simulink model "full_simulation_split_hil_new_connection"  (Simulink 7.9)
settings: Solver=ode1  StartTime=0  StopTime=10  FixedStep=Ts  RelTol=1e-8
values from neighbouring files (symbols this model uses):
  A_fx = 2e-2 * 0.4    (= 0.008)    [QR_DI_Init.m]    (also in quadro_cascade_disturbance_wo_wind.m)
  A_fy = A_fx    (= 0.008)    [QR_DI_Init.m]    (also in quadro_cascade_disturbance_wo_wind.m)
  A_fz = 2 * A_fx    (= 0.016)    [QR_DI_Init.m]    (also in quadro_cascade_disturbance_wo_wind.m)
  Bias_Phi = -0.0088    [QR_DI_Init.m]    (also in Reference_Calibration.m = mean(Phi))
  Bias_Theta = 0.022    [QR_DI_Init.m]    (also in Reference_Calibration.m = mean(Theta))
  command_on = 1    [QR_DI_Init.m]    (also in quadro_cascade_disturbance_wo_wind.m)
  cw_x = 1.05    [QR_DI_Init.m]    (also in quadro_cascade_disturbance_wo_wind.m)
  cw_y = cw_x    (= 1.05)    [QR_DI_Init.m]    (also in quadro_cascade_disturbance_wo_wind.m)
  cw_z = 1.05    [QR_DI_Init.m]    (also in quadro_cascade_disturbance_wo_wind.m)
  deltaTm = 0.2    [QR_DI_Init.m]    (also in quadro_cascade_disturbance_wo_wind.m)
  den_psi_ref = poly( ones(1,2) * -1 * T_psi_ref)    [QR_DI_Init.m]    (also in quadro_cascade_disturbance_wo_wind.m)
  den_x_ref = poly( ones(1,4) * -1 * T_x_ref)    [QR_DI_Init.m]    (also in quadro_cascade_disturbance_wo_wind.m)
  den_y_ref = poly( ones(1,4) * -1 * T_y_ref)    [QR_DI_Init.m]    (also in quadro_cascade_disturbance_wo_wind.m)
  den_z_ref = poly( ones(1,4) * -1 * T_z_ref)    [QR_DI_Init.m]    (also in quadro_cascade_disturbance_wo_wind.m)
  drot = 0.0117    [QR_DI_Init.m]    (also in quadro_cascade_disturbance_wo_wind.m = 0.2)
  dtran = 0.01    [QR_DI_Init.m]    (also in quadro_cascade_disturbance_wo_wind.m = 0.003)
  Fz_gain = 1 + 0.05*rand(1)    [QR_DI_Init.m]    (also in quadro_cascade_disturbance_wo_wind.m)
  Fz_lo = - 1.2 * m * g    (= -3.5316)    [QR_DI_Init.m]    (also in quadro_cascade_disturbance_wo_wind.m = -4.1202)
  Fz_up = 0    [QR_DI_Init.m]    (also in quadro_cascade_disturbance_wo_wind.m)
  g = 9.81    [QR_DI_Init.m]    (also in quadro_cascade_disturbance_wo_wind.m)
  Iq = [I_xx 0 0 ; 0 I_yy 0 ; 0 0 I_zz ]    [QR_DI_Init.m]    (also in quadro_cascade_disturbance_wo_wind.m = [0.0605 0 0; 0 0.0605 0; 0 0 0.018])
  K_err = old(:,2:end)    [QR_DI_Init.m]    (also in quadro_cascade_disturbance_wo_wind.m)
  K_Mot_Force = 0.3512    [QR_DI_Init.m]    (also in quadro_cascade_disturbance_wo_wind.m)
  K_Mot_Torque = 0.013    [QR_DI_Init.m]    (also in quadro_cascade_disturbance_wo_wind.m = 0.0013)
  l = 0.25    [QR_DI_Init.m]    (also in quadro_cascade_disturbance_wo_wind.m = 0.2775)
  m = 0.30    (= 0.3)    [QR_DI_Init.m]    (also in quadro_cascade_disturbance_wo_wind.m)
  m_real = m * ( 1 + 0.05*rand(1))    [QR_DI_Init.m]    (also in quadro_cascade_disturbance_wo_wind.m)
  Mm = 0.0    (= 0)    [QR_DI_Init.m]    (also in quadro_cascade_disturbance_wo_wind.m = 0.5)
  Mx_lo = - Mx_up    (= -0.2)    [QR_DI_Init.m]    (also in quadro_cascade_disturbance_wo_wind.m)
  Mx_up = 0.20    (= 0.2)    [QR_DI_Init.m]    (also in quadro_cascade_disturbance_wo_wind.m)
  My_lo = - My_up    (= -0.2)    [QR_DI_Init.m]    (also in quadro_cascade_disturbance_wo_wind.m)
  My_up = 0.20    (= 0.2)    [QR_DI_Init.m]    (also in quadro_cascade_disturbance_wo_wind.m)
  Mz_lo = - Mz_up    (= -0.02)    [QR_DI_Init.m]    (also in quadro_cascade_disturbance_wo_wind.m = -0.002)
  Mz_up = 0.02    [QR_DI_Init.m]    (also in quadro_cascade_disturbance_wo_wind.m = 0.002)
  phase_wind_z = 0    [QR_DI_Init.m]    (also in quadro_cascade_disturbance_wo_wind.m)
  psi_p_lim = 10*pi/180    (= 0.174532925199)    [QR_DI_Init.m]    (also in quadro_cascade_disturbance_wo_wind.m = 5)
  PWM_MAX = 200    [QR_DI_Init.m]    (also in quadro_cascade_disturbance_wo_wind.m)
  rho_air = 1.2041    [QR_DI_Init.m]    (also in quadro_cascade_disturbance_wo_wind.m)
  sample_time_noise_psi = 0.1    [QR_DI_Init.m]
  sample_time_noise_x = 0.2    [QR_DI_Init.m]
  sample_time_noise_y = 0.2    [QR_DI_Init.m]
  sample_time_noise_z = 0.1    [QR_DI_Init.m]
  seed_psi = seedvector(7)    [QR_DI_Init.m]
  seed_x = seedvector(1)    [QR_DI_Init.m]    (also in quadro_cascade_disturbance_wo_wind.m)
  seed_xp = seedvector(4)    [QR_DI_Init.m]    (also in quadro_cascade_disturbance_wo_wind.m)
  seed_y = seedvector(2)    [QR_DI_Init.m]    (also in quadro_cascade_disturbance_wo_wind.m)
  seed_yp = seedvector(5)    [QR_DI_Init.m]    (also in quadro_cascade_disturbance_wo_wind.m)
  seed_z = seedvector(3)    [QR_DI_Init.m]    (also in quadro_cascade_disturbance_wo_wind.m)
  seed_zp = seedvector(6)    [QR_DI_Init.m]    (also in quadro_cascade_disturbance_wo_wind.m)
  std_dev_psi = 1 * pi/180 * Noise_on    (= 0)    [QR_DI_Init.m]
  std_dev_x = 1e-1 * Noise_on    (= 0)    [QR_DI_Init.m]
  std_dev_xp = 0.03 * Noise_on    (= 0)    [QR_DI_Init.m]
  std_dev_y = 1e-1 * Noise_on    (= 0)    [QR_DI_Init.m]
  std_dev_yp = 0.03 * Noise_on    (= 0)    [QR_DI_Init.m]
  std_dev_z = 0.03 * Noise_on    (= 0)    [QR_DI_Init.m]
  std_dev_zp = 0.03 * Noise_on    (= 0)    [QR_DI_Init.m]
  T_refalt = 0.01    [QR_DI_Init.m]    (also in quadro_cascade_disturbance_wo_wind.m)
  T_wind_z = 24    [QR_DI_Init.m]    (also in quadro_cascade_disturbance_wo_wind.m)
  Tm = 10    [QR_DI_Init.m]    (also in quadro_cascade_disturbance_wo_wind.m)
  Ts = 1e-2    (= 0.01)    [QR_DI_Init.m]    (also in quadro_cascade_disturbance_wo_wind.m)
  v_wind_max_z = 2    [QR_DI_Init.m]    (also in quadro_cascade_disturbance_wo_wind.m)
  wind_on = 0    [QR_DI_Init.m]    (also in quadro_cascade_disturbance_wo_wind.m)
  x_p_lim = 1.5    [QR_DI_Init.m]    (also in quadro_cascade_disturbance_wo_wind.m = 5)
  y_p_lim = 1.5    [QR_DI_Init.m]    (also in quadro_cascade_disturbance_wo_wind.m = 5)
  z_p_lim = 1    [QR_DI_Init.m]    (also in quadro_cascade_disturbance_wo_wind.m = 1.5)
undefined symbols (not defined in the file or in its folder): T_wind_fine, v_wind_x_fine, v_wind_y_fine
libraries: simulink x5, dspsigops x4, Ports x4, aerolibtransform2 x3, dspmtrx3 x1, aerolibutil x1
(part 2 of 6)

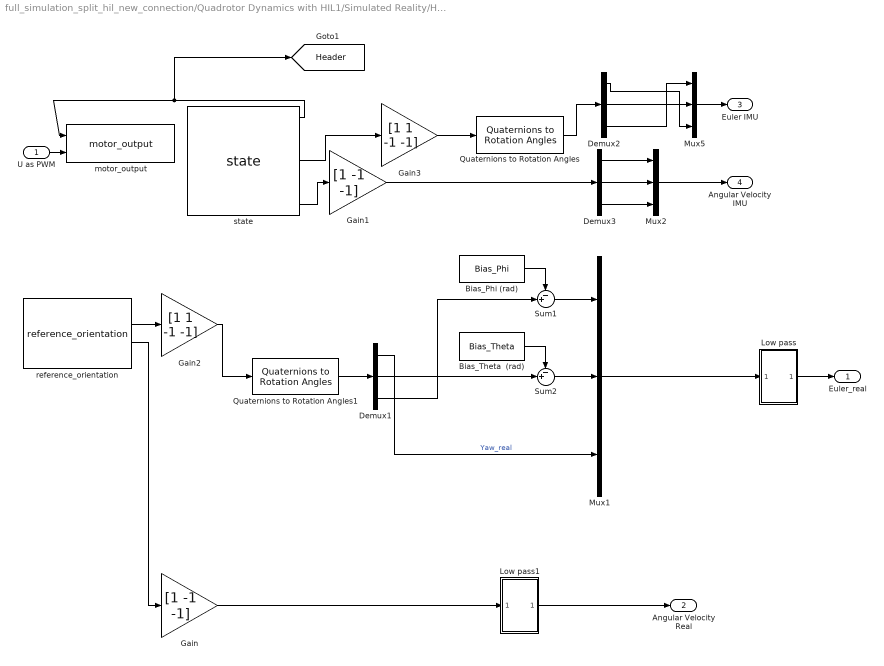
== system full_simulation_split_hil_new_connection/Quadrotor Dynamics with HIL1/Simulated Reality/HIL in the Loop for Rotation/Test Rig ==
  U as PWM : Inport
  Bias_Phi (rad) : Constant  Value=Bias_Phi
  Bias_Theta  (rad) : Constant  Value=Bias_Theta
  Demux1 : Demux  Outputs=3
  Demux2 : Demux  Outputs=3
  Demux3 : Demux  Outputs=3
  Gain : Gain  Gain=[1 -1 -1]
  Gain1 : Gain  Gain=[1 -1 -1]
  Gain2 : Gain  Gain=[1 1 -1 -1]
  Gain3 : Gain  Gain=[1 1 -1 -1]
  Low pass : Subsystem  mask{T_refalt=T_refalt}
  Low pass1 : Subsystem  mask{T_refalt=T_refalt}
  Mux1 : Mux  Inputs=3
  Mux2 : Mux  Inputs=3
  Mux5 : Mux  Inputs=3
  Quaternions to Rotation Angles : aerolibtransform2/Quaternions to Rotation Angles  rotationOrder=ZYX
  Quaternions to Rotation Angles1 : aerolibtransform2/Quaternions to Rotation Angles  rotationOrder=ZYX
  Sum1 : Sum  Inputs=-+|
  Sum2 : Sum  Inputs=-+|
  motor_output : Ports/motor_output
  reference_orientation : Ports/reference_orientation
  state : Ports/state
  "Euler_real " : Outport
  Angular Velocity Real : Outport  Port=2
  Euler IMU : Outport  Port=3
  Angular Velocity IMU : Outport  Port=4
  tag scope: Header=global
  wires:
  U as PWM/1 -> motor_output/2
  Mux5/1 -> Euler IMU/1
  Low pass/1(Out1) -> "Euler_real "/1
  state/1 -> motor_output/1, [Header]
  state/3 -> Gain3/1
  Quaternions to Rotation Angles/1 -> Demux2/1
  Demux2/2 -> Mux5/2
  Demux2/3 -> Mux5/1
  state/5 -> Gain1/1
  reference_orientation/2 -> Gain2/1
  reference_orientation/3 -> Gain/1
  Low pass1/1(Out1) -> Angular Velocity Real/1
  Gain2/1 -> Quaternions to Rotation Angles1/1
  Gain3/1 -> Quaternions to Rotation Angles/1
  Demux1/1 -> Mux1/3  "Yaw_real"
  Demux1/2 -> Sum2/2
  Quaternions to Rotation Angles1/1 -> Demux1/1
  Mux1/1 -> Low pass/1(In1)
  Gain/1 -> Low pass1/1(In1)
  Gain1/1 -> Demux3/1
  Demux3/1 -> Mux2/1
  Demux3/2 -> Mux2/2
  Mux2/1 -> Angular Velocity IMU/1
  Demux3/3 -> Mux2/3
  Demux2/1 -> Mux5/3
  Sum1/1 -> Mux1/1
  Sum2/1 -> Mux1/2
  Demux1/3 -> Sum1/2
  Bias_Phi (rad)/1 -> Sum1/1
  Bias_Theta  (rad)/1 -> Sum2/1

== system full_simulation_split_hil_new_connection/Quadrotor Dynamics with HIL1/Simulated Reality/Translation of the Quadrotor/transform to Inertial axes  ==
  x y z : Inport
  transform coefficients : Inport  Port=2
  Product : Product  Multiplication=Matrix(*)  SaturateOnIntegerOverflow=on  InputSameDT=on  OutDataTypeStr=Inherit: Same as first input
  Ve : Outport
  wires:
  x y z/1 -> Product/2
  transform coefficients/1 -> Product/1
  Product/1 -> Ve/1

== system full_simulation_split_hil_new_connection/Quadrotor Dynamics with HIL1/Simulated Reality/HIL in the Loop for Rotation/Test Rig/Low pass ==
  In1 : Inport
  Demux3 : Demux  Outputs=3
  Mux1 : Mux  Inputs=3
  Transfer Fcn1 : TransferFcn  Denominator=[T_refalt 1]
  Transfer Fcn2 : TransferFcn  Denominator=[T_refalt 1]
  Transfer Fcn3 : TransferFcn  Denominator=[T_refalt 1]
  Out1 : Outport
  wires:
  Demux3/1 -> Transfer Fcn1/1
  Transfer Fcn1/1 -> Mux1/1
  Demux3/2 -> Transfer Fcn2/1
  Transfer Fcn2/1 -> Mux1/2
  Demux3/3 -> Transfer Fcn3/1
  Transfer Fcn3/1 -> Mux1/3
  In1/1 -> Demux3/1
  Mux1/1 -> Out1/1

== system full_simulation_split_hil_new_connection/Quadrotor Dynamics with HIL1/Simulated Reality/HIL in the Loop for Rotation/Test Rig/Low pass1 ==
  In1 : Inport
  Demux3 : Demux  Outputs=3
  Mux1 : Mux  Inputs=3
  Transfer Fcn1 : TransferFcn  Denominator=[T_refalt 1]
  Transfer Fcn2 : TransferFcn  Denominator=[T_refalt 1]
  Transfer Fcn3 : TransferFcn  Denominator=[T_refalt 1]
  Out1 : Outport
  wires:
  Mux1/1 -> Out1/1
  In1/1 -> Demux3/1
  Transfer Fcn3/1 -> Mux1/3
  Demux3/3 -> Transfer Fcn3/1
  Transfer Fcn2/1 -> Mux1/2
  Demux3/2 -> Transfer Fcn2/1
  Transfer Fcn1/1 -> Mux1/1
  Demux3/1 -> Transfer Fcn1/1

== matlab function Dynamic Inversion of the Extended System/invAx SH/Embedded MATLAB Function ==
  data: xwhole_ext input double size=[14 1]; invAx output double size=[4 4]; m input double; I input double size=[3 3]; dtran input double; drot input double; Ax output double
function [invAx, Ax] = fcn(xwhole_ext, m, I, dtran, drot)
% This block supports the Embedded MATLAB subset.
% See the help menu for details. 
x = xwhole_ext(1);
y = xwhole_ext(2);
z = xwhole_ext(3);
dx = xwhole_ext(4);
dy = xwhole_ext(5);
dz = xwhole_ext(6);

phi = xwhole_ext(7);
theta = xwhole_ext(8);
psi = xwhole_ext(9);
p = xwhole_ext(10);
q = xwhole_ext(11);
r = xwhole_ext(12);

xi1 = xwhole_ext(13) +eps;
dxi1 = xwhole_ext(14) +eps;




% g = -9.81;  % not needed, S.H. 26.03.2013


Ixx = I(1,1);
Ixy = I(1,2);
Ixz = I(1,3);
Iyy = I(2,2);
Iyz = I(2,3);
Izz = I(3,3);

% invAx =[ ...
% (sin(phi)*sin(psi)*sin(theta)^2+cos(psi)*cos(phi)*sin(theta)+sin(psi)*cos(theta)^2*sin(phi))*m/(sin(psi)^2*sin(phi)^2*sin(theta)^2+sin(psi)^2*sin(phi)^2*cos(theta)^2+cos(psi)^2*cos(phi)^2*sin(theta)^2+cos(phi)^2*sin(psi)^2*sin(theta)^2+cos(psi)^2*sin(phi)^2*sin(theta)^2+cos(psi)^2*sin(phi)^2*cos(theta)^2+cos(theta)^2*cos(phi)^2*sin(psi)^2+cos(theta)^2*cos(phi)^2*cos(psi)^2),          -(-cos(phi)*sin(psi)*sin(theta)+cos(psi)*sin(phi)*sin(theta)^2+cos(psi)*cos(theta)^2*sin(phi))*m/(sin(psi)^2*sin(phi)^2*sin(theta)^2+sin(psi)^2*sin(phi)^2*cos(theta)^2+cos(psi)^2*cos(phi)^2*sin(theta)^2+cos(phi)^2*sin(psi)^2*sin(theta)^2+cos(psi)^2*sin(phi)^2*sin(theta)^2+cos(psi)^2*sin(phi)^2*cos(theta)^2+cos(theta)^2*cos(phi)^2*sin(psi)^2+cos(theta)^2*cos(phi)^2*cos(psi)^2),                                                                                                                                                                                                                                                                             cos(theta)*m*cos(phi)/(sin(phi)^2*sin(theta)^2+sin(phi)^2*cos(theta)^2+cos(theta)^2*cos(phi)^2+cos(phi)^2*sin(theta)^2),                                                                                                                                                                                                                                    sin(phi)*cos(phi)*sin(theta)*xi1*(sin(theta)^2+cos(theta)^2-1)/(sin(phi)^2*sin(theta)^2+sin(phi)^2*cos(theta)^2+cos(theta)^2*cos(phi)^2+cos(phi)^2*sin(theta)^2);...
% 1/xi1*(cos(phi)*sin(psi)*sin(theta)^2-cos(psi)*sin(phi)*sin(theta)+cos(theta)^2*cos(phi)*sin(psi))*m/(sin(psi)^2*sin(phi)^2*sin(theta)^2+sin(psi)^2*sin(phi)^2*cos(theta)^2+cos(psi)^2*cos(phi)^2*sin(theta)^2+cos(phi)^2*sin(psi)^2*sin(theta)^2+cos(psi)^2*sin(phi)^2*sin(theta)^2+cos(psi)^2*sin(phi)^2*cos(theta)^2+cos(theta)^2*cos(phi)^2*sin(psi)^2+cos(theta)^2*cos(phi)^2*cos(psi)^2)*Ixx, -1/xi1*(sin(phi)*sin(psi)*sin(theta)+cos(psi)*cos(phi)*sin(theta)^2+cos(theta)^2*cos(phi)*cos(psi))*m/(sin(psi)^2*sin(phi)^2*sin(theta)^2+sin(psi)^2*sin(phi)^2*cos(theta)^2+cos(psi)^2*cos(phi)^2*sin(theta)^2+cos(phi)^2*sin(psi)^2*sin(theta)^2+cos(psi)^2*sin(phi)^2*sin(theta)^2+cos(psi)^2*sin(phi)^2*cos(theta)^2+cos(theta)^2*cos(phi)^2*sin(psi)^2+cos(theta)^2*cos(phi)^2*cos(psi)^2)*Ixx,                                                                                                                                                                                                                                                                    -cos(theta)*Ixx*m*sin(phi)/(sin(phi)^2*sin(theta)^2+sin(phi)^2*cos(theta)^2+cos(theta)^2*cos(phi)^2+cos(phi)^2*sin(theta)^2)/xi1,                                         -(sin(phi)^2*cos(theta)^3*tan(theta)-sin(phi)^2*sin(theta)-cos(phi)^2*sin(theta)^3+sin(phi)^2*tan(theta)*cos(theta)*sin(theta)^2+cos(phi)^2*cos(theta)^3*tan(theta)+cos(theta)*tan(theta)*sin(theta)^2*cos(phi)^2-cos(theta)^2*cos(phi)^2*sin(theta))*Ixx/(sin(phi)^2*sin(theta)^2+sin(phi)^2*cos(theta)^2+cos(theta)^2*cos(phi)^2+cos(phi)^2*sin(theta)^2); ...
% 1/xi1*cos(psi)*m/(sin(psi)^2*sin(phi)^2*sin(theta)^2+sin(psi)^2*sin(phi)^2*cos(theta)^2+cos(psi)^2*cos(phi)^2*sin(theta)^2+cos(phi)^2*sin(psi)^2*sin(theta)^2+cos(psi)^2*sin(phi)^2*sin(theta)^2+cos(psi)^2*sin(phi)^2*cos(theta)^2+cos(theta)^2*cos(phi)^2*sin(psi)^2+cos(theta)^2*cos(phi)^2*cos(psi)^2)*Iyy*cos(theta),                                                                           1/xi1*sin(psi)*m/(sin(psi)^2*sin(phi)^2*sin(theta)^2+sin(psi)^2*sin(phi)^2*cos(theta)^2+cos(psi)^2*cos(phi)^2*sin(theta)^2+cos(phi)^2*sin(psi)^2*sin(theta)^2+cos(psi)^2*sin(phi)^2*sin(theta)^2+cos(psi)^2*sin(phi)^2*cos(theta)^2+cos(theta)^2*cos(phi)^2*sin(psi)^2+cos(theta)^2*cos(phi)^2*cos(psi)^2)*Iyy*cos(theta),                                                                                                                                                                                                                                                                             -sin(theta)*m*Iyy/(sin(phi)^2*sin(theta)^2+sin(phi)^2*cos(theta)^2+cos(theta)^2*cos(phi)^2+cos(phi)^2*sin(theta)^2)/xi1,                                                                                                                                                                                                                                             sin(phi)*(sin(theta)^2+cos(theta)^2-1)*Iyy*cos(theta)/(sin(phi)^2*sin(theta)^2+sin(phi)^2*cos(theta)^2+cos(theta)^2*cos(phi)^2+cos(phi)^2*sin(theta)^2) ;...
% -1/xi1*sin(phi)*cos(psi)*m/cos(phi)/(sin(psi)^2*sin(phi)^2*sin(theta)^2+sin(psi)^2*sin(phi)^2*cos(theta)^2+cos(psi)^2*cos(phi)^2*sin(theta)^2+cos(phi)^2*sin(psi)^2*sin(theta)^2+cos(psi)^2*sin(phi)^2*sin(theta)^2+cos(psi)^2*sin(phi)^2*cos(theta)^2+cos(theta)^2*cos(phi)^2*sin(psi)^2+cos(theta)^2*cos(phi)^2*cos(psi)^2)*cos(theta)*Izz,                                                        -1/xi1*sin(phi)*sin(psi)*m/cos(phi)/(sin(psi)^2*sin(phi)^2*sin(theta)^2+sin(psi)^2*sin(phi)^2*cos(theta)^2+cos(psi)^2*cos(phi)^2*sin(theta)^2+cos(phi)^2*sin(psi)^2*sin(theta)^2+cos(psi)^2*sin(phi)^2*sin(theta)^2+cos(psi)^2*sin(phi)^2*cos(theta)^2+cos(theta)^2*cos(phi)^2*sin(psi)^2+cos(theta)^2*cos(phi)^2*cos(psi)^2)*cos(theta)*Izz,                                                                                                                                                                                                                                                            sin(theta)*sin(phi)*m*Izz/(sin(phi)^2*sin(theta)^2+sin(phi)^2*cos(theta)^2+cos(theta)^2*cos(phi)^2+cos(phi)^2*sin(theta)^2)/xi1/cos(phi),                                                                                                                                                                                                              (sin(phi)^2+cos(phi)^2*sin(theta)^2+cos(theta)^2*cos(phi)^2)*cos(theta)*Izz/(sin(phi)^2*sin(theta)^2+sin(phi)^2*cos(theta)^2+cos(theta)^2*cos(phi)^2+cos(phi)^2*sin(theta)^2)/cos(phi);];
%
%
%
% Ax = [ ...
% 1/m*(sin(psi)*sin(phi)+cos(psi)*cos(phi)*sin(theta)),                                                                                                                                               xi1/m*(sin(psi)*cos(phi)-cos(psi)*sin(phi)*sin(theta))/Ixx,        (xi1/m*(sin(psi)*cos(phi)-cos(psi)*sin(phi)*sin(theta))*sin(phi)*tan(theta)+xi1/m*cos(psi)*cos(phi)^2*cos(theta)+xi1/m*(-cos(phi)*sin(psi)*sin(theta)+cos(psi)*sin(phi))*sin(phi)/cos(theta))/Iyy, (xi1/m*(sin(psi)*cos(phi)-cos(psi)*sin(phi)*sin(theta))*cos(phi)*tan(theta)-xi1/m*cos(psi)*cos(phi)*cos(theta)*sin(phi)+xi1/m*(-cos(phi)*sin(psi)*sin(theta)+cos(psi)*sin(phi))*cos(phi)/cos(theta))/Izz; ...
% 1/m*(cos(phi)*sin(psi)*sin(theta)-cos(psi)*sin(phi)),                                                                                                                                              xi1/m*(-sin(phi)*sin(psi)*sin(theta)-cos(psi)*cos(phi))/Ixx,        (xi1/m*(-sin(phi)*sin(psi)*sin(theta)-cos(psi)*cos(phi))*sin(phi)*tan(theta)+xi1/m*sin(psi)*cos(phi)^2*cos(theta)+xi1/m*(sin(psi)*sin(phi)+cos(psi)*cos(phi)*sin(theta))*sin(phi)/cos(theta))/Iyy, (xi1/m*(-sin(phi)*sin(psi)*sin(theta)-cos(psi)*cos(phi))*cos(phi)*tan(theta)-xi1/m*sin(psi)*cos(phi)*cos(theta)*sin(phi)+xi1/m*(sin(psi)*sin(phi)+cos(psi)*cos(phi)*sin(theta))*cos(phi)/cos(theta))/Izz; ...
% 1/m*cos(theta)*cos(phi),                                                                                                                                                                           -xi1/m*cos(theta)*sin(phi)/Ixx,                                                                                                                                (-xi1/m*cos(theta)*sin(phi)^2*tan(theta)-xi1/m*sin(theta)*cos(phi)^2)/Iyy,                                                                                                                  (-xi1/m*cos(theta)*sin(phi)*cos(phi)*tan(theta)+xi1/m*sin(theta)*cos(phi)*sin(phi))/Izz;...
% 0,                                                                                                                                                                                                        0,                                                                                                                                                                                  sin(phi)/cos(theta)/Iyy,                                                                                                                                                                                  cos(phi)/cos(theta)/Izz];
%      
% 
% 
% invAx = [...
%             (sin(phi)*sin(psi)*sin(theta)^2+cos(psi)*cos(phi)*sin(theta)+sin(psi)*cos(theta)^2*sin(phi))*m/(sin(psi)^2*sin(phi)^2*sin(theta)^2+sin(psi)^2*sin(phi)^2*cos(theta)^2+cos(psi)^2*cos(phi)^2*sin(theta)^2+cos(phi)^2*sin(psi)^2*sin(theta)^2+cos(psi)^2*sin(phi)^2*sin(theta)^2+cos(psi)^2*sin(phi)^2*cos(theta)^2+cos(phi)^2*cos(theta)^2*sin(psi)^2+cos(phi)^2*cos(theta)^2*cos(psi)^2),            (cos(phi)*sin(psi)*sin(theta)-cos(psi)*sin(phi)*sin(theta)^2-cos(psi)*cos(theta)^2*sin(phi))*m/(sin(psi)^2*sin(phi)^2*sin(theta)^2+sin(psi)^2*sin(phi)^2*cos(theta)^2+cos(psi)^2*cos(phi)^2*sin(theta)^2+cos(phi)^2*sin(psi)^2*sin(theta)^2+cos(psi)^2*sin(phi)^2*sin(theta)^2+cos(psi)^2*sin(phi)^2*cos(theta)^2+cos(phi)^2*cos(theta)^2*sin(psi)^2+cos(phi)^2*cos(theta)^2*cos(psi)^2),                                                                                                                                                                                                                                                                             cos(theta)*m*cos(phi)/(sin(phi)^2*sin(theta)^2+sin(phi)^2*cos(theta)^2+cos(phi)^2*sin(theta)^2+cos(phi)^2*cos(theta)^2),                                                                                                                                                                                                                                    sin(phi)*cos(phi)*sin(theta)*xi1*(sin(theta)^2+cos(theta)^2-1)/(sin(phi)^2*sin(theta)^2+sin(phi)^2*cos(theta)^2+cos(phi)^2*sin(theta)^2+cos(phi)^2*cos(theta)^2);...
%   1/xi1*(cos(phi)*sin(psi)*sin(theta)^2-cos(psi)*sin(phi)*sin(theta)+cos(theta)^2*cos(phi)*sin(psi))*m/(sin(psi)^2*sin(phi)^2*sin(theta)^2+sin(psi)^2*sin(phi)^2*cos(theta)^2+cos(psi)^2*cos(phi)^2*sin(theta)^2+cos(phi)^2*sin(psi)^2*sin(theta)^2+cos(psi)^2*sin(phi)^2*sin(theta)^2+cos(psi)^2*sin(phi)^2*cos(theta)^2+cos(phi)^2*cos(theta)^2*sin(psi)^2+cos(phi)^2*cos(theta)^2*cos(psi)^2)*Ixx, -1/xi1*(sin(phi)*sin(psi)*sin(theta)+cos(psi)*cos(phi)*sin(theta)^2+cos(theta)^2*cos(phi)*cos(psi))*m/(sin(psi)^2*sin(phi)^2*sin(theta)^2+sin(psi)^2*sin(phi)^2*cos(theta)^2+cos(psi)^2*cos(phi)^2*sin(theta)^2+cos(phi)^2*sin(psi)^2*sin(theta)^2+cos(psi)^2*sin(phi)^2*sin(theta)^2+cos(psi)^2*sin(phi)^2*cos(theta)^2+cos(phi)^2*cos(theta)^2*sin(psi)^2+cos(phi)^2*cos(theta)^2*cos(psi)^2)*Ixx,                                                                                                                                                                                                                                                                    -cos(theta)*Ixx*m*sin(phi)/(sin(phi)^2*sin(theta)^2+sin(phi)^2*cos(theta)^2+cos(phi)^2*sin(theta)^2+cos(phi)^2*cos(theta)^2)/xi1,                                         (-cos(phi)^2*sin(theta)^2*cos(theta)*tan(theta)-cos(phi)^2*cos(theta)^3*tan(theta)+cos(phi)^2*cos(theta)^2*sin(theta)+cos(phi)^2*sin(theta)^3-sin(phi)^2*cos(theta)^3*tan(theta)-sin(phi)^2*cos(theta)*tan(theta)*sin(theta)^2+sin(phi)^2*sin(theta))*Ixx/(sin(phi)^2*sin(theta)^2+sin(phi)^2*cos(theta)^2+cos(phi)^2*sin(theta)^2+cos(phi)^2*cos(theta)^2);...
%                                                                            1/xi1*cos(psi)*m/(sin(psi)^2*sin(phi)^2*sin(theta)^2+sin(psi)^2*sin(phi)^2*cos(theta)^2+cos(psi)^2*cos(phi)^2*sin(theta)^2+cos(phi)^2*sin(psi)^2*sin(theta)^2+cos(psi)^2*sin(phi)^2*sin(theta)^2+cos(psi)^2*sin(phi)^2*cos(theta)^2+cos(phi)^2*cos(theta)^2*sin(psi)^2+cos(phi)^2*cos(theta)^2*cos(psi)^2)*Iyy*cos(theta),                                                                           1/xi1*sin(psi)*m/(sin(psi)^2*sin(phi)^2*sin(theta)^2+sin(psi)^2*sin(phi)^2*cos(theta)^2+cos(psi)^2*cos(phi)^2*sin(theta)^2+cos(phi)^2*sin(psi)^2*sin(theta)^2+cos(psi)^2*sin(phi)^2*sin(theta)^2+cos(psi)^2*sin(phi)^2*cos(theta)^2+cos(phi)^2*cos(theta)^2*sin(psi)^2+cos(phi)^2*cos(theta)^2*cos(psi)^2)*Iyy*cos(theta),                                                                                                                                                                                                                                                                             -sin(theta)*m*Iyy/(sin(phi)^2*sin(theta)^2+sin(phi)^2*cos(theta)^2+cos(phi)^2*sin(theta)^2+cos(phi)^2*cos(theta)^2)/xi1,                                                                                                                                                                                                                                             sin(phi)*(sin(theta)^2+cos(theta)^2-1)*Iyy*cos(theta)/(sin(phi)^2*sin(theta)^2+sin(phi)^2*cos(theta)^2+cos(phi)^2*sin(theta)^2+cos(phi)^2*cos(theta)^2);...
%                                                         -1/xi1*sin(phi)*cos(psi)*m/cos(phi)/(sin(psi)^2*sin(phi)^2*sin(theta)^2+sin(psi)^2*sin(phi)^2*cos(theta)^2+cos(psi)^2*cos(phi)^2*sin(theta)^2+cos(phi)^2*sin(psi)^2*sin(theta)^2+cos(psi)^2*sin(phi)^2*sin(theta)^2+cos(psi)^2*sin(phi)^2*cos(theta)^2+cos(phi)^2*cos(theta)^2*sin(psi)^2+cos(phi)^2*cos(theta)^2*cos(psi)^2)*cos(theta)*Izz,                                                        -1/xi1*sin(phi)*sin(psi)*m/cos(phi)/(sin(psi)^2*sin(phi)^2*sin(theta)^2+sin(psi)^2*sin(phi)^2*cos(theta)^2+cos(psi)^2*cos(phi)^2*sin(theta)^2+cos(phi)^2*sin(psi)^2*sin(theta)^2+cos(psi)^2*sin(phi)^2*sin(theta)^2+cos(psi)^2*sin(phi)^2*cos(theta)^2+cos(phi)^2*cos(theta)^2*sin(psi)^2+cos(phi)^2*cos(theta)^2*cos(psi)^2)*cos(theta)*Izz,                                                                                                                                                                                                                                                            sin(theta)*sin(phi)*m*Izz/(sin(phi)^2*sin(theta)^2+sin(phi)^2*cos(theta)^2+cos(phi)^2*sin(theta)^2+cos(phi)^2*cos(theta)^2)/xi1/cos(phi),                                                                                                                                                                                                              (cos(phi)^2*cos(theta)^2+sin(phi)^2+cos(phi)^2*sin(theta)^2)*cos(theta)*Izz/(sin(phi)^2*sin(theta)^2+sin(phi)^2*cos(theta)^2+cos(phi)^2*sin(theta)^2+cos(phi)^2*cos(theta)^2)/cos(phi)];
%  
%  
%  

% S.H. 26.03.2013
Ax =    [ (sin(phi)*sin(psi) + cos(phi)*cos(psi)*sin(theta))/m,  (xi1*(cos(phi)*sin(psi) - cos(psi)*sin(phi)*sin(theta)))/(Ixx*m), ((xi1*sin(phi)*(cos(psi)*sin(phi) - cos(phi)*sin(psi)*sin(theta)))/(m*cos(theta)) + (xi1*cos(phi)^2*cos(psi)*cos(theta))/m + (xi1*sin(phi)*tan(theta)*(cos(phi)*sin(psi) - cos(psi)*sin(phi)*sin(theta)))/m)/Iyy,  ((xi1*cos(phi)*(cos(psi)*sin(phi) - cos(phi)*sin(psi)*sin(theta)))/(m*cos(theta)) + (xi1*cos(phi)*tan(theta)*(cos(phi)*sin(psi) - cos(psi)*sin(phi)*sin(theta)))/m - (xi1*cos(phi)*cos(psi)*cos(theta)*sin(phi))/m)/Izz;
         -(cos(psi)*sin(phi) - cos(phi)*sin(psi)*sin(theta))/m, -(xi1*(cos(phi)*cos(psi) + sin(phi)*sin(psi)*sin(theta)))/(Ixx*m), ((xi1*sin(phi)*(sin(phi)*sin(psi) + cos(phi)*cos(psi)*sin(theta)))/(m*cos(theta)) + (xi1*cos(phi)^2*cos(theta)*sin(psi))/m - (xi1*sin(phi)*tan(theta)*(cos(phi)*cos(psi) + sin(phi)*sin(psi)*sin(theta)))/m)/Iyy, -((xi1*cos(phi)*tan(theta)*(cos(phi)*cos(psi) + sin(phi)*sin(psi)*sin(theta)))/m - (xi1*cos(phi)*(sin(phi)*sin(psi) + cos(phi)*cos(psi)*sin(theta)))/(m*cos(theta)) + (xi1*cos(phi)*cos(theta)*sin(phi)*sin(psi))/m)/Izz;
                                       (cos(phi)*cos(theta))/m,                                -(xi1*cos(theta)*sin(phi))/(Ixx*m),                                                                                                                                  -((xi1*cos(phi)^2*sin(theta))/m + (xi1*cos(theta)*sin(phi)^2*tan(theta))/m)/Iyy,                                                                                                                             ((xi1*cos(phi)*sin(phi)*sin(theta))/m - (xi1*cos(phi)*cos(theta)*sin(phi)*tan(theta))/m)/Izz;
                                                             0,                                                                 0,                                                                                                                                                                                        sin(phi)/(Iyy*cos(theta)),                                                                                                                                                                                                cos(phi)/(Izz*cos(theta))];
 

invAx = [  m*sin(phi)*sin(psi) + m*cos(phi)*cos(psi)*sin(theta),            m*cos(phi)*sin(psi)*sin(theta) - m*cos(psi)*sin(phi),                      m*cos(phi)*cos(theta),                         0;
 (Ixx*m*(cos(phi)*sin(psi) - cos(psi)*sin(phi)*sin(theta)))/xi1, -(Ixx*m*(cos(phi)*cos(psi) + sin(phi)*sin(psi)*sin(theta)))/xi1,           -(Ixx*m*cos(theta)*sin(phi))/xi1,                         0;
                                (Iyy*m*cos(psi)*cos(theta))/xi1,                                 (Iyy*m*cos(theta)*sin(psi))/xi1,                    -(Iyy*m*sin(theta))/xi1,                         0;
           -(Izz*m*cos(psi)*cos(theta)*sin(phi))/(xi1*cos(phi)),            -(Izz*m*cos(theta)*sin(phi)*sin(psi))/(xi1*cos(phi)), (Izz*m*sin(phi)*sin(theta))/(xi1*cos(phi)), (Izz*cos(theta))/cos(phi)];
